simulink model "step_test"  (R2022a)
settings: Solver=ode45  StartTime=0.0  StopTime=360  RelTol=1e-3  EnableMultiTasking=on
libraries: arduino_io_lib x8
settings Model: Creator=Gabriel  LastModifiedBy=PC
settings SolverCC: AlgebraicLoopSolver=TrustRegion
settings DataIOCC: LimitDataPoints=on  SaveFormat=Array  ReturnWorkspaceOutputs=off
settings OptimizationCC: LifeSpan=inf
settings DebuggingCC: UnderspecifiedInitializationDetection=Classic  MergeDetectMultiDrivingBlocksExec=none  SolverPrmCheckMsg=warning  UnconnectedInputMsg=warning  UnconnectedOutputMsg=warning  UnconnectedLineMsg=warning  StateNameClashWarn=warning  SFUnexpectedBacktrackingDiag=warning  SFNoUnconditionalDefaultTransitionDiag=warning  SFExecutionAtInitializationDiag=none  SFMachineParentedDataDiag=warning  ArithmeticOperatorsInVariantConditions=warning
settings HardwareCC: ProdBitPerPointer=32  ProdBitPerSizeT=32  ProdBitPerPtrDiffT=32  ProdLargestAtomicFloat=None  ProdIntDivRoundTo=Undefined  ProdEndianess=Unspecified  ProdWordSize=32  ProdHWDeviceType=32-bit Generic
settings ModelReferenceCC: PropagateSignalLabelsOutOfModel=off
settings SFSimCC: SimUseLocalCustomCode=off  CustomCodeUndefinedFunction=UseInterfaceOnly
settings RTWCC: RTWUseLocalCustomCode=off
settings CodeAppCC: StateflowObjectComments=on
settings GRTTargetCC: TargetLangStandard=C89/C90 (ANSI)
settings ConfigComp: CovMetricSettings=dw  CovSaveCumulativeToWorkspaceVar=on  CovSaveSingleToWorkspaceVar=on  CovExternalEMLEnable=off

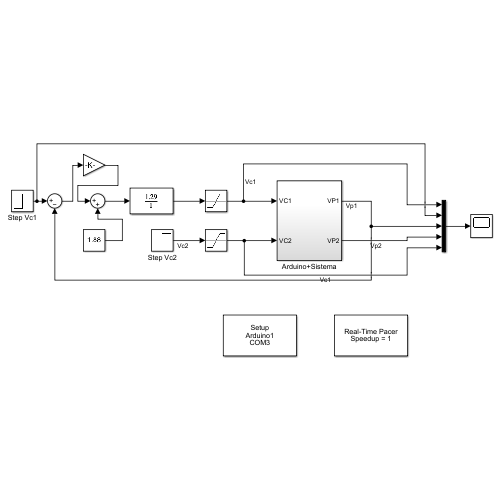
[thumbnail: Simulink's stored preview of the top-level diagram]
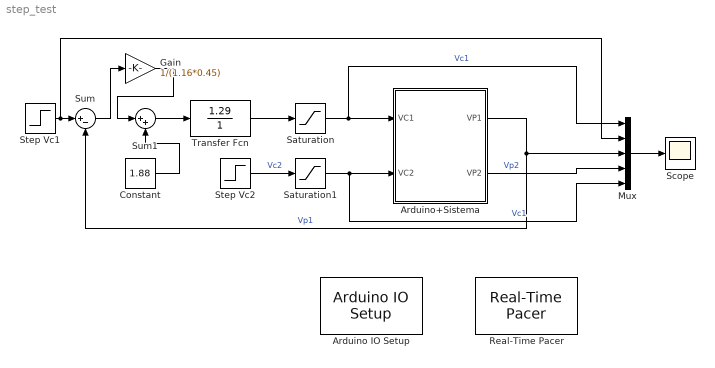
== system step_test ==
  Arduino IO Setup : arduino_io_lib/Arduino IO Setup  Priority=3  arduinoVar=Temporary arduino variable: Arduino1  workspaceVarName=a  comPort=COM3
  Arduino+Sistema : Subsystem
  Constant : Constant  Value=1.88
  Gain : Gain  Gain=1/(1.16*0.45)
  Mux : Mux  Inputs=5
  Real-Time Pacer : arduino_io_lib/Real-Time Pacer  simTimePerRealTime=1
  Saturation : Saturate  UpperLimit=5  LowerLimit=0
  Saturation1 : Saturate  UpperLimit=5  LowerLimit=0
  Scope : Scope
  Step Vc1 : Step  After=3.26  SampleTime=0
  Step Vc2 : Step  Time=20  SampleTime=0
  Sum : Sum  Inputs=|+-
  Sum1 : Sum  Inputs=|++
  Transfer Fcn : TransferFcn  Numerator=[1.29]  Denominator=[0 1]
  wires:
  Saturation/1 -> Arduino+Sistema/1(VC1), Mux/1  "Vc1"
  Mux/1 -> Scope/1
  Arduino+Sistema/1(VP1) -> Sum/2, Mux/3  "Vp1"
  Arduino+Sistema/2(VP2) -> Mux/4  "Vp2"
  Step Vc2/1 -> Saturation1/1  "Vc2"
  Saturation1/1 -> Mux/5, Arduino+Sistema/2(VC2)  "Vc1"
  Transfer Fcn/1 -> Saturation/1
  Step Vc1/1 -> Mux/2, Sum/1
  Sum/1 -> Gain/1
  Constant/1 -> Sum1/2
  Gain/1 -> Sum1/1
  Sum1/1 -> Transfer Fcn/1

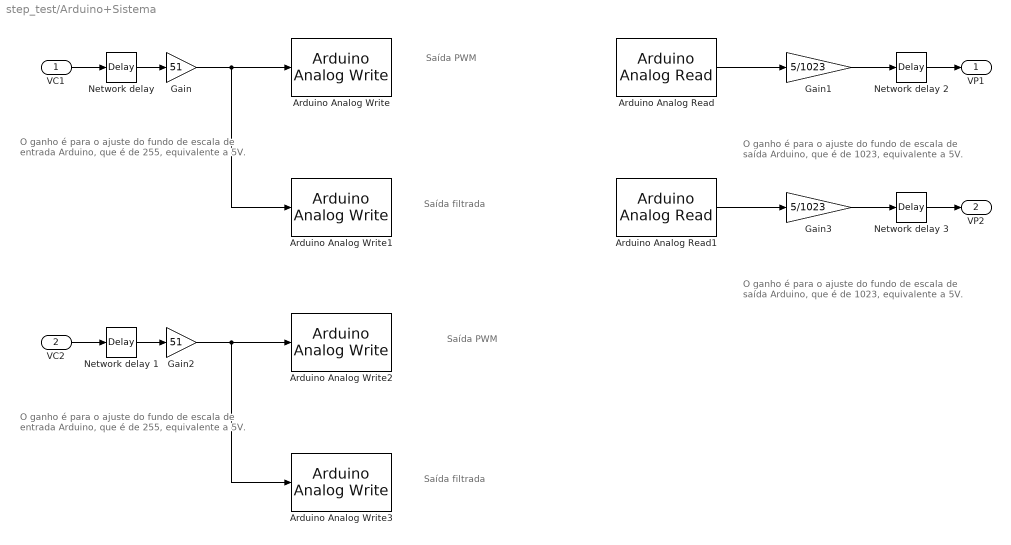
== system step_test/Arduino+Sistema ==
  note: Saída PWM
  note: O ganho é para o ajuste do fundo de escala
      | de saída Arduino, que é de 1023, equivalente
      | a 5V.
  note: O ganho é para o ajuste do fundo de escala
      | de entrada Arduino, que é de 255, equivalente
      | a 5V.
  note: Saída filtrada
  note: O ganho é para o ajuste do fundo de escala
      | de saída Arduino, que é de 1023, equivalente
      | a 5V.
  note: Saída PWM
  note: O ganho é para o ajuste do fundo de escala
      | de entrada Arduino, que é de 255, equivalente
      | a 5V.
  note: Saída filtrada
  VC1 : Inport
  VC2 : Inport  Port=2
  Arduino Analog Read : arduino_io_lib/Arduino Analog Read  arduinoVar=Temporary arduino variable: Arduino1  arduinoPin=0  T=0.02
  Arduino Analog Read1 : arduino_io_lib/Arduino Analog Read  arduinoVar=Temporary arduino variable: Arduino1  arduinoPin=1  T=0.02
  Arduino Analog Write : arduino_io_lib/Arduino Analog Write  arduinoVar=Temporary arduino variable: Arduino1  arduinoPin=11  T=0.02
  Arduino Analog Write1 : arduino_io_lib/Arduino Analog Write  arduinoVar=Temporary arduino variable: Arduino1  arduinoPin=5  T=0.02
  Arduino Analog Write2 : arduino_io_lib/Arduino Analog Write  arduinoVar=Temporary arduino variable: Arduino1  arduinoPin=3  T=0.02
  Arduino Analog Write3 : arduino_io_lib/Arduino Analog Write  arduinoVar=Temporary arduino variable: Arduino1  arduinoPin=6  T=0.02
  Gain : Gain  Gain=51
  Gain1 : Gain  Gain=5/1023
  Gain2 : Gain  Gain=51
  Gain3 : Gain  Gain=5/1023
  Network delay {,1..3} (4 alike) : TransportDelay  DelayTime=0
  VP1 : Outport  VectorParamsAs1DForOutWhenUnconnected=off
  VP2 : Outport  Port=2  VectorParamsAs1DForOutWhenUnconnected=off
  wires:
  VC1/1 -> "Network delay "/1
  Arduino Analog Read/1 -> Gain1/1
  Gain1/1 -> Network delay 2/1
  "Network delay "/1 -> Gain/1
  Network delay 2/1 -> VP1/1
  Gain/1 -> Arduino Analog Write/1, Arduino Analog Write1/1
  Arduino Analog Read1/1 -> Gain3/1
  Gain3/1 -> Network delay 3/1
  Network delay 3/1 -> VP2/1
  VC2/1 -> Network delay 1/1
  Network delay 1/1 -> Gain2/1
  Gain2/1 -> Arduino Analog Write2/1, Arduino Analog Write3/1
